simulink model "rtwdemo_secondOrderSystem"  (R2017b)
settings: Solver=ode3  StartTime=0.0  StopTime=.2  FixedStep=0.001  RelTol=1e-3  EnableMultiTasking=on
settings Model: SimulationMode=external  Creator=The MathWorks, Inc.  LastModifiedBy=EIB
settings DataIOCC: SaveFormat=StructureWithTime  SaveState=on  InspectSignalLogs=on  SignalLoggingName=logsOut
settings OptimizationCC: UseFloatMulNetSlope=on  EnhancedBackFolding=on  ExpressionDepthLimit=2147483647  EfficientFloat2IntCast=on  LifeSpan=inf
settings DebuggingCC: SaveWithParameterizedLinksMsg=none  UnderspecifiedInitializationDetection=Classic  MergeDetectMultiDrivingBlocksExec=none  CheckExecutionContextPreStartOutputMsg=on  CheckExecutionContextRuntimeOutputMsg=on  SignalResolutionControl=TryResolveAllWithWarning  MultiTaskDSMMsg=warning  MultiTaskCondExecSysMsg=none  AllowSymbolicDim=off  StateNameClashWarn=warning  SFUnexpectedBacktrackingDiag=warning  SFNoUnconditionalDefaultTransitionDiag=warning  SFExecutionAtInitializationDiag=none
settings ModelReferenceCC: PropagateSignalLabelsOutOfModel=off
settings RTWCC: Description=Generic Real-Time Target  GenerateReport=on  RTWVerbose=off  BuildConfiguration=Faster Runs  LaunchReport=on  CheckMdlBeforeBuild=Warning
settings CodeAppCC: ForceParamTrailComments=on  StateflowObjectComments=on
settings GRTTargetCC: TargetLangStandard=C89/C90 (ANSI)  UtilityFuncGeneration=Shared location  GeneratePreprocessorConditionals=Disable all
settings ConfigComp: CovMetricSettings=dw  CovHtmlReporting=on  CovSaveCumulativeToWorkspaceVar=on  CovSaveSingleToWorkspaceVar=on  CovExternalEMLEnable=off

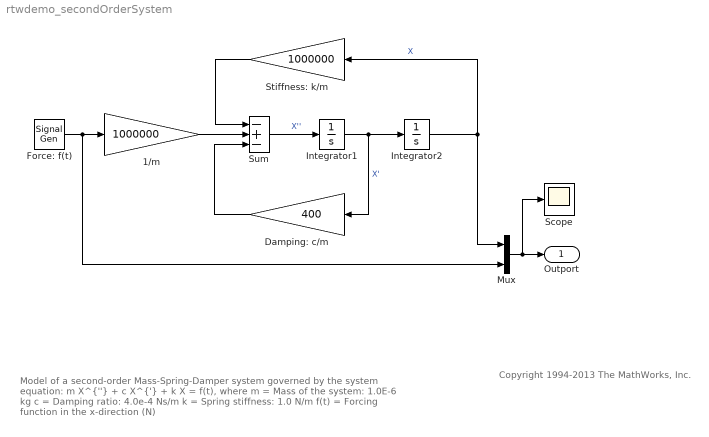
== system rtwdemo_secondOrderSystem ==
  note: Copyright 1994-2013 The MathWorks, Inc.
  note: Model of a second-order Mass-Spring-Damper system
      | governed by the system equation:
      |
      | m X^{''} + c X^{'} + k X = f(t), where
      |
      | m   = Mass of the system: 1.0E-6 kg
      | c    = Damping ratio: 4.0e-4 Ns/m
      | k    = Spring stiffness: 1.0 N/m
      | f(t) = Forcing function in the x-direction (N)
  1/m : Gain  Gain=1000000  SaturateOnIntegerOverflow=on  OutDataTypeStr=Inherit: Same as input  ParamDataTypeStr=Inherit: Same as input
  Damping: c/m : Gain  Gain=400  SaturateOnIntegerOverflow=on  OutDataTypeStr=Inherit: Same as input  ParamDataTypeStr=Inherit: Same as input
  Force: f(t) : SignalGenerator  WaveForm=square  Amplitude=4  Frequency=20
  Integrator1 : Integrator
  Integrator2 : Integrator
  Mux : Mux  Inputs=2
  Scope : Scope
  Stiffness: k/m : Gain  Gain=1000000  SaturateOnIntegerOverflow=on  OutDataTypeStr=Inherit: Same as input  ParamDataTypeStr=Inherit: Same as input
  Sum : Sum  Inputs=-+-  SaturateOnIntegerOverflow=on  InputSameDT=on  OutDataTypeStr=Inherit: Same as first input
  Outport : Outport  InitialOutput=0
  wires:
  Stiffness: k/m/1 -> Sum/1
  Integrator1/1 -> Integrator2/1, Damping: c/m/1  "X'"
  Integrator2/1 -> Mux/1, Stiffness: k/m/1  "X"
  Damping: c/m/1 -> Sum/3
  Mux/1 -> Scope/1, Outport/1
  1/m/1 -> Sum/2
  Sum/1 -> Integrator1/1  "X''"
  Force: f(t)/1 -> 1/m/1, Mux/2
